simulink model "sps2se_pvinverter_avg"  (R2014a)
settings: Solver=ode15s  StartTime=0.0  StopTime=1  FixedStep=Ts  MaxStep=1e-3  RelTol=1e-4
PreLoadFcn:
  | PVArrayIsc = 5;
  | PVArrayVoc = 21.6;
  | PVArrayRs = 0.036;
  | Tcircuit = 27.15;
  | Toffset = -2;
  | TIPH1 = 0.001;
  | TXIS1 = 3;
  | TRS1 = 0;
  | Ts = 1e-4;
InitFcn:
  | Ts = 1e-4;
StartFcn:
  | tic;
StopFcn:
  | toc;
undefined symbols (not defined in the file or in its folder): sigbuilder_block
libraries: elec_lib x37, powerlib x9, nesl_utility x4, fl_lib x3, powerlib_meascontrol x1
settings Model: Creator=cosorio  LastModifiedBy=cosorio
settings DataIOCC: LimitDataPoints=off  SignalLoggingSaveFormat=ModelDataLogs  SaveOutput=off  SignalLogging=off  SaveTime=off
settings OptimizationCC: ExpressionDepthLimit=2147483647
settings DebuggingCC: UnderspecifiedInitializationDetection=Classic  SolverPrmCheckMsg=none  FcnCallInpInsideContextMsg=UseLocalSettings  StateNameClashWarn=warning
settings GRTTargetCC: CombineOutputUpdateFcns=off  GRTInterface=on

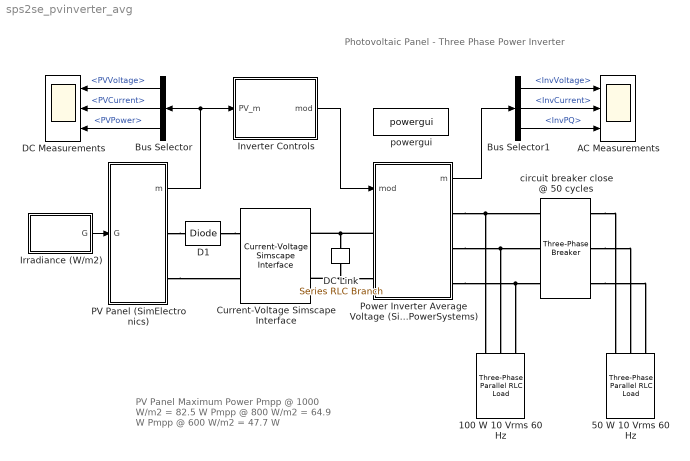
== system sps2se_pvinverter_avg ==
  note: Photovoltaic Panel - Three Phase Power Inverter
  note: PV Panel Maximum Power
      | Pmpp @ 1000 W/m2 = 82.5 W
      | Pmpp @ 800 W/m2 = 64.9 W
      | Pmpp @ 600 W/m2 = 47.7 W
  100 W 10 Vrms 60 Hz : powerlib/Elements/Three-Phase Parallel RLC Load  LConnTagsString=A|B|C  Configuration=Y (grounded)  NominalVoltage=10  NominalFrequency=60  ActivePower=100  InductivePower=0  CapacitivePower=0  Measurements=None  LoadType=constant Z
  50 W 10 Vrms 60 Hz : powerlib/Elements/Three-Phase Parallel RLC Load  LConnTagsString=A|B|C  Configuration=Y (grounded)  NominalVoltage=10  NominalFrequency=60  ActivePower=50  InductivePower=0  CapacitivePower=0  Measurements=None  LoadType=constant Z
  AC Measurements : Scope  NumInputPorts=3
      settings: YMin=-10~-10~0  YMax=10~10~100  SaveName=InverterData
  Bus Selector : BusSelector  OutputSignals=PVVoltage,PVCurrent,PVPower
  Bus Selector1 : BusSelector  OutputSignals=InvVoltage,InvCurrent,InvPQ
  Current-Voltage Simscape Interface : powerlib/Interface Elements/Current-Voltage Simscape Interface  DFT=off  FMode=Unit delay (discrete)  T=1e-4  Ts=1e-4  i0=0  v0=18  Sd=SimPowerSystems side  Measurements=off
  D1 : elec_lib/Semiconductor Devices/Diode  ModelType=3  Vf=0.6 V  Ron=0.3 Ohm  Goff=1e-8 S  Rz=0.3 Ohm  Vz=50 V  C_PWL=5 pF  prmExp=1  I12=[ 0.0137 0.545 ] A  V12=[ 0.6 0.7 ] V  I1=0.0137 A  V1=0.6 V  RS=0.01 Ohm  IS=1e-12 A  Tmeas=25 C  ec=1  BV=Inf V  C_param=1  CJ0=5 pF  VJ=1 V  Mgrad=0.5  Vvec=[ 0.1 10 100 ] V  Cvec=[ 3.5 1 0.4 ] pF  FC=0.5  Q_param=1  Irrm=-7.15 A  iF=4 A  didt=-750 A/us  trr=115 ns  TT=50 ns  tau=100 ns  T_param=1  IS_T2=1.25e-7 A  I1_T2=0.245 A  V1_T2=0.5 V  Tmeas2=125 C  EG_param=1  EG=1.11 eV  XTI_param=1  XTI=3  dBVdT=0 V/K  Tdevice=25 C  Rth=[ 0 10 ] K/W  thermal_mass_parameterization=1  thermal_mass=[ 0 1 ] J/K  thermal_time_constant=[ 0 10 ] s  thermal_mass_initial_temperatures=[ 25 25 ] C
  DC Link : powerlib/Elements/Series RLC Branch  LConnTagsString=__new0  RConnTagsString=__new0  BranchType=C  Resistance=1  Inductance=1e-3  SetiL0=off  InitialCurrent=0  Capacitance=480e-6  Setx0=on  InitialVoltage=18  Measurements=None
  DC Measurements : Scope  NumInputPorts=3
      settings: YMin=0~0~0  YMax=25~6~100
  Inverter Controls : Subsystem  TreatAsAtomicUnit=on  SystemSampleTime=1e-4
  Irradiance (W/m2) : Subsystem  Tag=STV Subsys  LoadFcn=sigbuilder_block('load');  StartFcn=sigbuilder_block('start');  StopFcn=sigbuilder_block('stop');  ClipboardFcn=sigbuilder_block('clipboard');  mask(Sigbuilder block){}
      mask help: Sigbuilder GUI
      mask init:
      | if ~strcmp(get_param(bdroot(gcbh),'SimulationStatus'),'stopped') tuvar = sigbuilder_block('maskInit'); end
      settings: CopyFcn=sigbuilder_block('copy');  DeleteFcn=sigbuilder_block('delete');  ModelCloseFcn=sigbuilder_block('modelClose');  PreSaveFcn=sigbuilder_block('preSave');  PauseFcn=sigbuilder_block('pause')  ContinueFcn=sigbuilder_block('continue')  NameChangeFcn=sigbuilder_block('namechange');  OpenFcn=sigbuilder_block('open',[124.138 46.5517 550.552 391.034 ]);  CloseFcn=sigbuilder_block('close');
      mask Display: plot(0,0,100,100,[10,10,40,40,10],[80,20,20,80,80],[40,10],[50,50], [40,27,10],[65,72,56],[40,25,25,10],[28,28,43,43]);
  PV Panel (SimElectronics) : Subsystem
  Power Inverter Average Voltage (SimPowerSystems) : Subsystem
  circuit breaker close @ 50 cycles : powerlib/Elements/Three-Phase Breaker  InitialState=open  SwitchA=on  SwitchB=on  SwitchC=on  SwitchTimes=[50/60]  External=off  BreakerResistance=0.001  SnubberResistance=1e6  SnubberCapacitance=inf  Measurements=None
  powergui : powerlib/powergui  Priority=1  SimulationMode=Discrete  SolverType=Tustin  SampleTime=Ts  frequency=60  SPID=off  DisableSnubberDevices=off  DisableRonSwitches=off  DisableVfSwitches=off  SwTol=0  Interpol=off  DisplayEquations=off  Ts=0  methode=off  frequencyindice=0  Pbase=100e6  ErrMax=1e-4  Iterations=50  UnitsV=kV  UnitsW=MW  FunctionMessages=off  echomessages=off  HookPort=off  EnableUseOfTLC=off  x0status=blocks  RestoreLinks=warning  ResistiveCurrentMeasurement=off  Frange=[0:2:500]  Ylog=off  Xlog=on  ShowGrid=off  save=off  variable=ZData  structure=0  ZoomFFT=on  StartTime=0.0  cycles=1  DisplayStyle=1  fundamental=60  FreqAxis=off  MaxFrequency=1000  frequencyindicesteady=1  RmsSteady=1  display=off
  wires:
  Irradiance (W/m2)/1(G) -> PV Panel (SimElectronics)/1(G)
  PV Panel (SimElectronics)/1(m) -> Bus Selector/1, Inverter Controls/1(PV_m)
  Bus Selector/3 -> DC Measurements/3  "<PVPower>"
  Bus Selector/1 -> DC Measurements/1  "<PVVoltage>"
  Bus Selector/2 -> DC Measurements/2  "<PVCurrent>"
  Power Inverter Average Voltage (SimPowerSystems)/1(m) -> Bus Selector1/1
  Bus Selector1/1 -> AC Measurements/1  "<InvVoltage>"
  Bus Selector1/2 -> AC Measurements/2  "<InvCurrent>"
  Bus Selector1/3 -> AC Measurements/3  "<InvPQ>"
  Inverter Controls/1(mod) -> Power Inverter Average Voltage (SimPowerSystems)/1(mod)
  connections:
  PV Panel (SimElectronics)/RConn2 -- Current-Voltage Simscape Interface/RConn2
  DC Link/RConn1 -- Current-Voltage Simscape Interface/LConn2 -- Power Inverter Average Voltage (SimPowerSystems)/LConn2
  Power Inverter Average Voltage (SimPowerSystems)/LConn1 -- Current-Voltage Simscape Interface/LConn1 -- DC Link/LConn1
  PV Panel (SimElectronics)/RConn1 -- D1/LConn1
  D1/RConn1 -- Current-Voltage Simscape Interface/RConn1
  Power Inverter Average Voltage (SimPowerSystems)/RConn1 -- 100 W 10 Vrms 60 Hz/LConn1 -- circuit breaker close @ 50 cycles/LConn1
  Power Inverter Average Voltage (SimPowerSystems)/RConn3 -- 100 W 10 Vrms 60 Hz/LConn3 -- circuit breaker close @ 50 cycles/LConn3
  Power Inverter Average Voltage (SimPowerSystems)/RConn2 -- 100 W 10 Vrms 60 Hz/LConn2 -- circuit breaker close @ 50 cycles/LConn2
  circuit breaker close @ 50 cycles/RConn1 -- 50 W 10 Vrms 60 Hz/LConn1
  circuit breaker close @ 50 cycles/RConn2 -- 50 W 10 Vrms 60 Hz/LConn2
  circuit breaker close @ 50 cycles/RConn3 -- 50 W 10 Vrms 60 Hz/LConn3

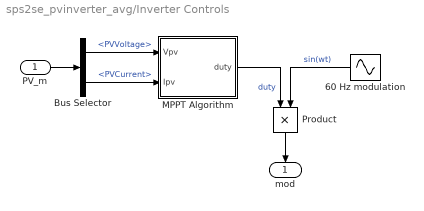
== system sps2se_pvinverter_avg/Inverter Controls ==
  PV_m : Inport
  60 Hz modulation : Sin  Frequency=2*pi*60  Phase=[0, 120*pi/180, -120*pi/180]  SampleTime=1e-4
  Bus Selector : BusSelector  OutputSignals=PVVoltage,PVCurrent
  MPPT Algorithm : Subsystem
  Product : Product  RndMeth=Zero
  mod : Outport
  wires:
  60 Hz modulation/1 -> Product/2  "sin(wt)"
  PV_m/1 -> Bus Selector/1
  Product/1 -> mod/1
  Bus Selector/1 -> MPPT Algorithm/1(Vpv)  "<PVVoltage>"
  Bus Selector/2 -> MPPT Algorithm/2(Ipv)  "<PVCurrent>"
  MPPT Algorithm/1(duty) -> Product/1  "duty"

== system sps2se_pvinverter_avg/Irradiance (W//m2) ==
  Demux : Demux  Tag=STV Demux  Outputs=1
  FromWs : FromWorkspace  Tag=STV FromWs  VariableName=tuvar  SampleTime=0
      SigBuilderData=|
      | common.afterFinalStr = 'Extrapolate'
      | common.sampleTime = '0'
      | dataSet(1).timeRange = [0 1]
      | dataSet(1).name = 'Constant Irradiance'
      | dataSet(2).timeRange = [0 1]
      | dataSet(2).name = 'Step Irradiance'
      | dataSet(3).timeRange = [0 1]
      | dataSet(3).name = 'Trapezoidal Irradiance'
      | sbobj.Groups(1).Name = 'Constant Irradiance'
      | sbobj.Groups(1).Signals.Name = 'G'
      | sbobj.Groups(1).Signals.XData = [0 1]
      | sbobj.Groups(1).Signals.YData = [800 800]
      | sbobj.Groups(1).TimeRange = [0 1]
      | sbobj.Groups(2).Name = 'Step Irradiance'
      | sbobj.Groups(2).Signals.Name = 'G'
      | sbobj.Groups(2).Signals.XData = [0 0.5 0.5 1]
      | sbobj.Groups(2).Signals.YData = [600 600 1000 1000]
      | sbobj.Groups(2).TimeRange = [0 1]
      | sbobj.Groups(3).Name = 'Trapezoidal Irradiance'
      | sbobj.Groups(3).Signals.Name = 'G'
      | sbobj.Groups(3).Signals.XData = [0 0.2 0.3 0.5 0.7 0.9 1]
      | sbobj.Groups(3).Signals.YData = [800 800 600 600 1000 1000 800]
      | sbobj.Groups(3).TimeRange = [0 1]
  G : Outport  Tag=STV Outport
  wires:
  Demux/1 -> G/1
  FromWs/1 -> Demux/1

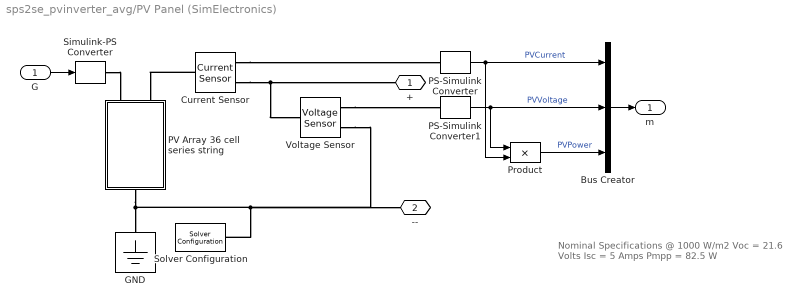
== system sps2se_pvinverter_avg/PV Panel (SimElectronics) ==
  note: Nominal Specifications @ 1000 W/m2
      | Voc = 21.6 Volts
      | Isc = 5 Amps
      | Pmpp = 82.5 W
  G : Inport
  Bus Creator : BusCreator  Inputs=3
  Current Sensor : fl_lib/Electrical/Electrical Sensors/Current Sensor
  GND : fl_lib/Electrical/Electrical Elements/Electrical Reference
  PS-Simulink Converter : nesl_utility/PS-Simulink Converter  PhysicalDomain=network_engine_domain  SubClassName=ps_output  LeftPortType=input  RightPortType=output  PseudoPeriodic=off  Frequencies=[]  Unit=A  AffineConversion=off
  PS-Simulink Converter1 : nesl_utility/PS-Simulink Converter  PhysicalDomain=network_engine_domain  SubClassName=ps_output  LeftPortType=input  RightPortType=output  PseudoPeriodic=off  Frequencies=[]  Unit=V  AffineConversion=off
  PV Array 36 cell series string : Subsystem
  Product : Product  RndMeth=Zero
  Simulink-PS Converter : nesl_utility/Simulink-PS Converter  PhysicalDomain=network_engine_domain  SubClassName=ps_input  LeftPortType=input  RightPortType=output  PseudoPeriodic=off  Frequencies=[]  NoiseDistribution=none  NoiseParameters=[]  Unit=W/m^2  AffineConversion=off  InputFiltering=off  SimscapeFilterOrder=1  InputFilterTimeConstant=1e-4  UdotUserProvided=0
  Solver Configuration : nesl_utility/Solver Configuration  PhysicalDomain=network_engine_domain  SubClassName=solver  LeftPortType=input  RightPortType=generic  Accelerate=off  Tones=[]  Harmonics=[]  SimulateNoise=off  Profile=off  UseLocalSampling=off  EnableSwitchedLinearOptims=on  FrequencyDomain=off  UseCCode=off  RelTol=0.001  AbsTol=1e-06  MinStep=1e-09  ToWorkspace=off  DoDC=on  ResidualTolerance=1e-9  UseLocalSolver=on  LocalSolverChoice=NE_BACKWARD_EULER_ADVANCER  LocalSolverSampleTime=1e-4  DoFixedCost=on  MaxNonlinIter=4  MaxModeIter=2  LinearAlgebra=Sparse  DelaysMemoryBudget=1024  AutomaticFiltering=on  FilteringTimeConstant=0.001
  Voltage Sensor : fl_lib/Electrical/Electrical Sensors/Voltage Sensor
  + : PMIOPort  Port=1  Side=Right
  -- : PMIOPort  Port=2  Side=Right
  m : Outport
  wires:
  G/1 -> Simulink-PS Converter/1
  PS-Simulink Converter/1 -> Bus Creator/1, Product/2  "PVCurrent"
  PS-Simulink Converter1/1 -> Bus Creator/2, Product/1  "PVVoltage"
  Bus Creator/1 -> m/1
  Product/1 -> Bus Creator/3  "PVPower"
  connections:
  --/RConn1 -- Voltage Sensor/RConn2 -- Solver Configuration/RConn1 -- PV Array 36 cell series string/RConn1 -- GND/LConn1
  Simulink-PS Converter/RConn1 -- PV Array 36 cell series string/LConn1
  Current Sensor/LConn1 -- PV Array 36 cell series string/LConn2
  Current Sensor/RConn2 -- +/RConn1 -- Voltage Sensor/LConn1
  Current Sensor/RConn1 -- PS-Simulink Converter/LConn1
  Voltage Sensor/RConn1 -- PS-Simulink Converter1/LConn1

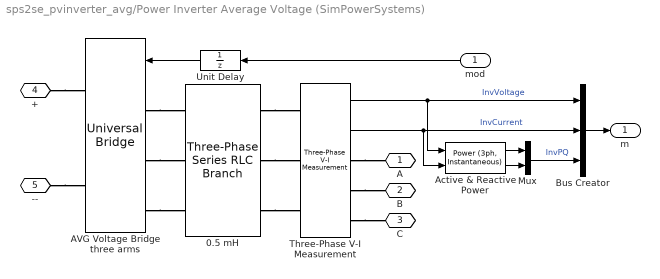
== system sps2se_pvinverter_avg/Power Inverter Average Voltage (SimPowerSystems) ==
  mod : Inport
  0.5 mH : powerlib/Elements/Three-Phase Series RLC Branch  LConnTagsString=A|B|C  RConnTagsString=A|B|C  BranchType=L  Resistance=1.0  Inductance=500e-6  Capacitance=1.0  Measurements=None
  AVG Voltage Bridge three arms : powerlib/Power Electronics/Universal Bridge  Arms=3  SnubberResistance=1e5  SnubberCapacitance=inf  Device=Average-model based VSC  Ron=1e-3  Lon=0  ForwardVoltages="[  0  0  ]"  ForwardVoltage=0  GTOparameters=[ 10e-6 , 20e-6 ]  IGBTparameters=[ 1e-6 , 2e-6 ]  Measurements=None  Measurements_2=None  converterType=Rectifier
  Active & Reactive Power : powerlib_meascontrol/Measurements/Power (3ph, Instantaneous)
  Bus Creator : BusCreator  Inputs=3
  Mux : Mux  Inputs=2
  Three-Phase V-I Measurement : powerlib/Measurements/Three-Phase V-I Measurement  VoltageMeasurement=phase-to-ground  SetLabelV=off  LabelV=Vabc  Vpu=off  VpuLL=off  CurrentMeasurement=yes  SetLabelI=off  LabelI=Iabc  Ipu=off  Pbase=100e6  Vbase=500e3  OutputType=Complex  PhasorSimulation=off  PSBequivalent=0
  Unit Delay : UnitDelay  SampleTime=Ts
  A : PMIOPort  Port=1  Side=Right
  B : PMIOPort  Port=2  Side=Right
  C : PMIOPort  Port=3  Side=Right
  + : PMIOPort  Port=4  Side=Left
  -- : PMIOPort  Port=5  Side=Left
  m : Outport
  wires:
  Three-Phase V-I Measurement/1 -> Bus Creator/1, Active & Reactive Power/1  "InvVoltage"
  Mux/1 -> Bus Creator/3  "InvPQ"
  Three-Phase V-I Measurement/2 -> Bus Creator/2, Active & Reactive Power/2  "InvCurrent"
  Bus Creator/1 -> m/1
  mod/1 -> Unit Delay/1
  Unit Delay/1 -> AVG Voltage Bridge three arms/1
  Active & Reactive Power/2 -> Mux/2
  Active & Reactive Power/1 -> Mux/1
  connections:
  AVG Voltage Bridge three arms/LConn1 -- 0.5 mH/LConn1
  AVG Voltage Bridge three arms/LConn2 -- 0.5 mH/LConn2
  AVG Voltage Bridge three arms/LConn3 -- 0.5 mH/LConn3
  0.5 mH/RConn1 -- Three-Phase V-I Measurement/LConn1
  0.5 mH/RConn2 -- Three-Phase V-I Measurement/LConn2
  0.5 mH/RConn3 -- Three-Phase V-I Measurement/LConn3
  Three-Phase V-I Measurement/RConn1 -- A/RConn1
  Three-Phase V-I Measurement/RConn2 -- B/RConn1
  Three-Phase V-I Measurement/RConn3 -- C/RConn1
  +/RConn1 -- AVG Voltage Bridge three arms/RConn1
  --/RConn1 -- AVG Voltage Bridge three arms/RConn2

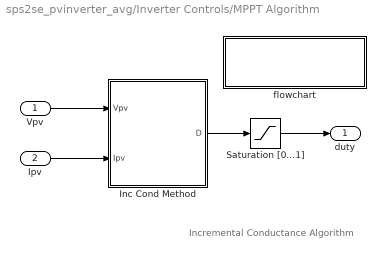
== system sps2se_pvinverter_avg/Inverter Controls/MPPT Algorithm ==
  note: Incremental Conductance Algorithm
  Vpv : Inport  OutDataTypeStr=double  PortDimensions=1  SampleTime=[0.0001,0]
  Ipv : Inport  Port=2  OutDataTypeStr=double  PortDimensions=1  SampleTime=[0.0001,0]
  Inc Cond Method : Stateflow chart  TreatAsAtomicUnit=on
  Saturation [0...1] : Saturate  UpperLimit=1  LowerLimit=0
  flowchart : Subsystem
      settings: OpenFcn=winopen('INC.jpg');
      mask Display: disp('Algorithm\nFlowchart')
  duty : Outport  OutDataTypeStr=double  PortDimensions=1  SampleTime=[0.0001,0]
  wires:
  Inc Cond Method/1(D) -> Saturation [0...1]/1
  Vpv/1 -> Inc Cond Method/1(Vpv)
  Ipv/1 -> Inc Cond Method/2(Ipv)
  Saturation [0...1]/1 -> duty/1

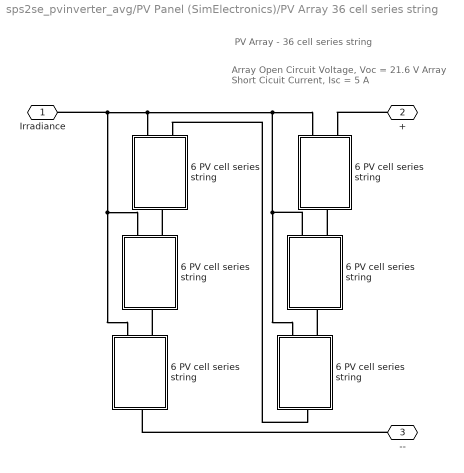
== system sps2se_pvinverter_avg/PV Panel (SimElectronics)/PV Array 36 cell series string ==
  note: Array Open Circuit Voltage, Voc = 21.6 V
      | Array Short Cicuit Current, Isc = 5 A
  note: PV Array - 36 cell series string
  6 PV cell series string : Subsystem  mask(PV String){Isc=PVArrayIsc, Voc=PVArrayVoc/6, N=1.5, Rs=PVArrayRs/6, TIPH1=TIPH1, TXIS1=TXIS1, TRS1=TRS1, TOFFSET=Toffset}
      mask prompts: Isc "Short-circuit current (A) :"; Voc "Open-circuit voltage (V) :"; N "Quality factor :"; Rs "Series resistance (ohms) :"; TIPH1 "1st order temperature coefficient for solar generated current (1/oC) :"; TXIS1 "Temperature exponent for diode saturation current :"; TRS1 "Temperature exponent for series resistance :"; TOFFSET "Offset local circuit temperature (oC) :"
      mask help:
      | PV series string.
      | This block models six (6) photo-voltaic cells connected in series.
      | The base parameters are measured at an irradiance of 1000 W/m2 and a device
      | temperature of 25oC.
      | The string short-circuit current is equal to the short-circuit current of each
      | individual cell.
      | The string open-circuit voltage is equal to six times the open-circuit voltage
      | of each individual cell.
      | The string series resistance is equal to six times the series resistance of
      | each individual cell.
      | The offset local circuit temperature is the difference between the string
      | temperature and the specified circuit temperature.
  "6 PV cell series string " : Subsystem  mask(PV String){Isc=PVArrayIsc, Voc=PVArrayVoc/6, N=1.5, Rs=PVArrayRs/6, TIPH1=TIPH1, TXIS1=TXIS1, TRS1=TRS1, TOFFSET=Toffset}
      mask prompts: Isc "Short-circuit current (A) :"; Voc "Open-circuit voltage (V) :"; N "Quality factor :"; Rs "Series resistance (ohms) :"; TIPH1 "1st order temperature coefficient for solar generated current (1/oC) :"; TXIS1 "Temperature exponent for diode saturation current :"; TRS1 "Temperature exponent for series resistance :"; TOFFSET "Offset local circuit temperature (oC) :"
      mask help:
      | PV series string.
      | This block models six (6) photo-voltaic cells connected in series.
      | The base parameters are measured at an irradiance of 1000 W/m2 and a device
      | temperature of 25oC.
      | The string short-circuit current is equal to the short-circuit current of each
      | individual cell.
      | The string open-circuit voltage is equal to six times the open-circuit voltage
      | of each individual cell.
      | The string series resistance is equal to six times the series resistance of
      | each individual cell.
      | The offset local circuit temperature is the difference between the string
      | temperature and the specified circuit temperature.
  "6 PV cell series string  " : Subsystem  mask(PV String){Isc=PVArrayIsc, Voc=PVArrayVoc/6, N=1.5, Rs=PVArrayRs/6, TIPH1=TIPH1, TXIS1=TXIS1, TRS1=TRS1, TOFFSET=Toffset}
      mask prompts: Isc "Short-circuit current (A) :"; Voc "Open-circuit voltage (V) :"; N "Quality factor :"; Rs "Series resistance (ohms) :"; TIPH1 "1st order temperature coefficient for solar generated current (1/oC) :"; TXIS1 "Temperature exponent for diode saturation current :"; TRS1 "Temperature exponent for series resistance :"; TOFFSET "Offset local circuit temperature (oC) :"
      mask help:
      | PV series string.
      | This block models six (6) photo-voltaic cells connected in series.
      | The base parameters are measured at an irradiance of 1000 W/m2 and a device
      | temperature of 25oC.
      | The string short-circuit current is equal to the short-circuit current of each
      | individual cell.
      | The string open-circuit voltage is equal to six times the open-circuit voltage
      | of each individual cell.
      | The string series resistance is equal to six times the series resistance of
      | each individual cell.
      | The offset local circuit temperature is the difference between the string
      | temperature and the specified circuit temperature.
  "6 PV cell series string   " : Subsystem  mask(PV String){Isc=PVArrayIsc, Voc=PVArrayVoc/6, N=1.5, Rs=PVArrayRs/6, TIPH1=TIPH1, TXIS1=TXIS1, TRS1=TRS1, TOFFSET=Toffset}
      mask prompts: Isc "Short-circuit current (A) :"; Voc "Open-circuit voltage (V) :"; N "Quality factor :"; Rs "Series resistance (ohms) :"; TIPH1 "1st order temperature coefficient for solar generated current (1/oC) :"; TXIS1 "Temperature exponent for diode saturation current :"; TRS1 "Temperature exponent for series resistance :"; TOFFSET "Offset local circuit temperature (oC) :"
      mask help:
      | PV series string.
      | This block models six (6) photo-voltaic cells connected in series.
      | The base parameters are measured at an irradiance of 1000 W/m2 and a device
      | temperature of 25oC.
      | The string short-circuit current is equal to the short-circuit current of each
      | individual cell.
      | The string open-circuit voltage is equal to six times the open-circuit voltage
      | of each individual cell.
      | The string series resistance is equal to six times the series resistance of
      | each individual cell.
      | The offset local circuit temperature is the difference between the string
      | temperature and the specified circuit temperature.
  "6 PV cell series string    " : Subsystem  mask(PV String){Isc=PVArrayIsc, Voc=PVArrayVoc/6, N=1.5, Rs=PVArrayRs/6, TIPH1=TIPH1, TXIS1=TXIS1, TRS1=TRS1, TOFFSET=Toffset}
      mask prompts: Isc "Short-circuit current (A) :"; Voc "Open-circuit voltage (V) :"; N "Quality factor :"; Rs "Series resistance (ohms) :"; TIPH1 "1st order temperature coefficient for solar generated current (1/oC) :"; TXIS1 "Temperature exponent for diode saturation current :"; TRS1 "Temperature exponent for series resistance :"; TOFFSET "Offset local circuit temperature (oC) :"
      mask help:
      | PV series string.
      | This block models six (6) photo-voltaic cells connected in series.
      | The base parameters are measured at an irradiance of 1000 W/m2 and a device
      | temperature of 25oC.
      | The string short-circuit current is equal to the short-circuit current of each
      | individual cell.
      | The string open-circuit voltage is equal to six times the open-circuit voltage
      | of each individual cell.
      | The string series resistance is equal to six times the series resistance of
      | each individual cell.
      | The offset local circuit temperature is the difference between the string
      | temperature and the specified circuit temperature.
  "6 PV cell series string     " : Subsystem  mask(PV String){Isc=PVArrayIsc, Voc=PVArrayVoc/6, N=1.5, Rs=PVArrayRs/6, TIPH1=TIPH1, TXIS1=TXIS1, TRS1=TRS1, TOFFSET=Toffset}
      mask prompts: Isc "Short-circuit current (A) :"; Voc "Open-circuit voltage (V) :"; N "Quality factor :"; Rs "Series resistance (ohms) :"; TIPH1 "1st order temperature coefficient for solar generated current (1/oC) :"; TXIS1 "Temperature exponent for diode saturation current :"; TRS1 "Temperature exponent for series resistance :"; TOFFSET "Offset local circuit temperature (oC) :"
      mask help:
      | PV series string.
      | This block models six (6) photo-voltaic cells connected in series.
      | The base parameters are measured at an irradiance of 1000 W/m2 and a device
      | temperature of 25oC.
      | The string short-circuit current is equal to the short-circuit current of each
      | individual cell.
      | The string open-circuit voltage is equal to six times the open-circuit voltage
      | of each individual cell.
      | The string series resistance is equal to six times the series resistance of
      | each individual cell.
      | The offset local circuit temperature is the difference between the string
      | temperature and the specified circuit temperature.
  Irradiance : PMIOPort  Port=1  Side=Left
  + : PMIOPort  Port=2  Side=Left
  -- : PMIOPort  Port=3  Side=Right
  connections:
  "6 PV cell series string    "/LConn1 -- "6 PV cell series string     "/LConn1 -- Irradiance/RConn1 -- "6 PV cell series string  "/LConn1 -- "6 PV cell series string "/LConn1 -- 6 PV cell series string/LConn1 -- "6 PV cell series string   "/LConn1
  --/RConn1 -- "6 PV cell series string     "/RConn1
  +/RConn1 -- 6 PV cell series string/LConn2
  "6 PV cell series string     "/LConn2 -- "6 PV cell series string    "/RConn1
  "6 PV cell series string    "/LConn2 -- "6 PV cell series string   "/RConn1
  "6 PV cell series string  "/RConn1 -- "6 PV cell series string   "/LConn2
  "6 PV cell series string  "/LConn2 -- "6 PV cell series string "/RConn1
  "6 PV cell series string "/LConn2 -- 6 PV cell series string/RConn1

== system sps2se_pvinverter_avg/Inverter Controls/MPPT Algorithm/flowchart ==

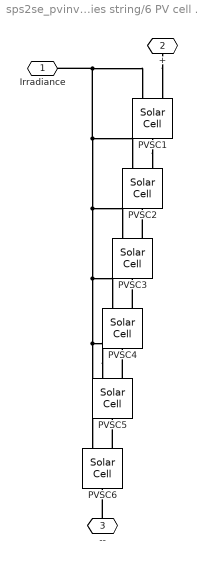
== system sps2se_pvinverter_avg/PV Panel (SimElectronics)/PV Array 36 cell series string/6 PV cell series string ==
  PVSC{1..6} (6 alike) : elec_lib/Sources/Solar Cell  prm=1  Isc=Isc A  Voc=Voc/6 V  Is=1e-06 A  Is2=0 A  Iph=7.34 A  Ir0=1000 W/m^2  ec=N  N2=2  Rs=Rs/6 Ohm  Rp=Inf Ohm  N_series=1  TIPH1=TIPH1 1/K  EG=1.11 eV  TXIS1=TXIS1  TXIS2=3  TRS1=TRS1  TRP1=0  Tmeas=25 C  TFIXED=25 C  thermal_mass=100 J/K  initial_temperature=25 C
  Irradiance : PMIOPort  Port=1  Side=Left
  + : PMIOPort  Port=2  Side=Left
  -- : PMIOPort  Port=3  Side=Right
  connections:
  --/RConn1 -- PVSC6/RConn1
  +/RConn1 -- PVSC1/LConn2
  PVSC6/LConn2 -- PVSC5/RConn1
  PVSC5/LConn2 -- PVSC4/RConn1
  PVSC4/LConn2 -- PVSC3/RConn1
  PVSC3/LConn2 -- PVSC2/RConn1
  PVSC1/RConn1 -- PVSC2/LConn2
  PVSC5/LConn1 -- PVSC4/LConn1 -- PVSC3/LConn1 -- PVSC2/LConn1 -- PVSC1/LConn1 -- Irradiance/RConn1 -- PVSC6/LConn1

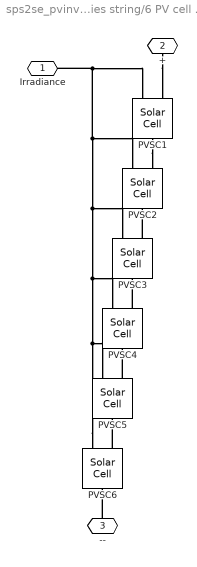
== system sps2se_pvinverter_avg/PV Panel (SimElectronics)/PV Array 36 cell series string/6 PV cell series string  ==
  PVSC{1..6} (6 alike) : elec_lib/Sources/Solar Cell  prm=1  Isc=Isc A  Voc=Voc/6 V  Is=1e-06 A  Is2=0 A  Iph=7.34 A  Ir0=1000 W/m^2  ec=N  N2=2  Rs=Rs/6 Ohm  Rp=Inf Ohm  N_series=1  TIPH1=TIPH1 1/K  EG=1.11 eV  TXIS1=TXIS1  TXIS2=3  TRS1=TRS1  TRP1=0  Tmeas=25 C  TFIXED=25 C  thermal_mass=100 J/K  initial_temperature=25 C
  Irradiance : PMIOPort  Port=1  Side=Left
  + : PMIOPort  Port=2  Side=Left
  -- : PMIOPort  Port=3  Side=Right
  connections:
  PVSC6/LConn1 -- Irradiance/RConn1 -- PVSC1/LConn1 -- PVSC2/LConn1 -- PVSC3/LConn1 -- PVSC4/LConn1 -- PVSC5/LConn1
  PVSC1/RConn1 -- PVSC2/LConn2
  PVSC3/LConn2 -- PVSC2/RConn1
  PVSC4/LConn2 -- PVSC3/RConn1
  PVSC5/LConn2 -- PVSC4/RConn1
  PVSC6/LConn2 -- PVSC5/RConn1
  +/RConn1 -- PVSC1/LConn2
  --/RConn1 -- PVSC6/RConn1

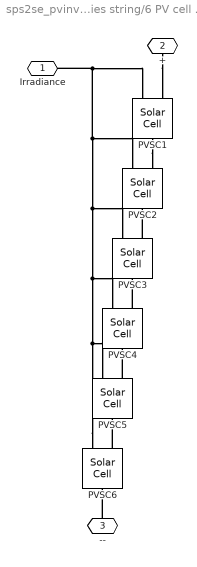
== system sps2se_pvinverter_avg/PV Panel (SimElectronics)/PV Array 36 cell series string/6 PV cell series string   ==
  PVSC{1..6} (6 alike) : elec_lib/Sources/Solar Cell  prm=1  Isc=Isc A  Voc=Voc/6 V  Is=1e-06 A  Is2=0 A  Iph=7.34 A  Ir0=1000 W/m^2  ec=N  N2=2  Rs=Rs/6 Ohm  Rp=Inf Ohm  N_series=1  TIPH1=TIPH1 1/K  EG=1.11 eV  TXIS1=TXIS1  TXIS2=3  TRS1=TRS1  TRP1=0  Tmeas=25 C  TFIXED=25 C  thermal_mass=100 J/K  initial_temperature=25 C
  Irradiance : PMIOPort  Port=1  Side=Left
  + : PMIOPort  Port=2  Side=Left
  -- : PMIOPort  Port=3  Side=Right
  connections:
  PVSC6/LConn1 -- Irradiance/RConn1 -- PVSC1/LConn1 -- PVSC2/LConn1 -- PVSC3/LConn1 -- PVSC4/LConn1 -- PVSC5/LConn1
  PVSC1/RConn1 -- PVSC2/LConn2
  PVSC3/LConn2 -- PVSC2/RConn1
  PVSC4/LConn2 -- PVSC3/RConn1
  PVSC5/LConn2 -- PVSC4/RConn1
  PVSC6/LConn2 -- PVSC5/RConn1
  +/RConn1 -- PVSC1/LConn2
  --/RConn1 -- PVSC6/RConn1

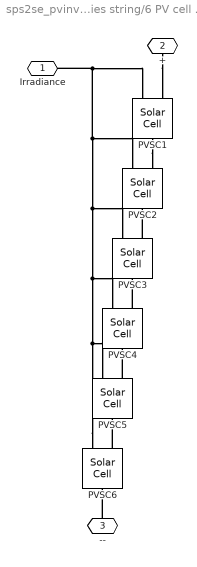
== system sps2se_pvinverter_avg/PV Panel (SimElectronics)/PV Array 36 cell series string/6 PV cell series string    ==
  PVSC{1..6} (6 alike) : elec_lib/Sources/Solar Cell  prm=1  Isc=Isc A  Voc=Voc/6 V  Is=1e-06 A  Is2=0 A  Iph=7.34 A  Ir0=1000 W/m^2  ec=N  N2=2  Rs=Rs/6 Ohm  Rp=Inf Ohm  N_series=1  TIPH1=TIPH1 1/K  EG=1.11 eV  TXIS1=TXIS1  TXIS2=3  TRS1=TRS1  TRP1=0  Tmeas=25 C  TFIXED=25 C  thermal_mass=100 J/K  initial_temperature=25 C
  Irradiance : PMIOPort  Port=1  Side=Left
  + : PMIOPort  Port=2  Side=Left
  -- : PMIOPort  Port=3  Side=Right
  connections:
  PVSC6/LConn1 -- Irradiance/RConn1 -- PVSC1/LConn1 -- PVSC2/LConn1 -- PVSC3/LConn1 -- PVSC4/LConn1 -- PVSC5/LConn1
  PVSC1/RConn1 -- PVSC2/LConn2
  PVSC3/LConn2 -- PVSC2/RConn1
  PVSC4/LConn2 -- PVSC3/RConn1
  PVSC5/LConn2 -- PVSC4/RConn1
  PVSC6/LConn2 -- PVSC5/RConn1
  +/RConn1 -- PVSC1/LConn2
  --/RConn1 -- PVSC6/RConn1

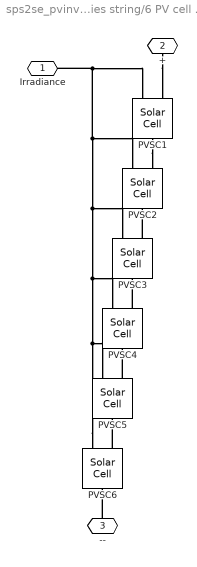
== system sps2se_pvinverter_avg/PV Panel (SimElectronics)/PV Array 36 cell series string/6 PV cell series string     ==
  PVSC{1..6} (6 alike) : elec_lib/Sources/Solar Cell  prm=1  Isc=Isc A  Voc=Voc/6 V  Is=1e-06 A  Is2=0 A  Iph=7.34 A  Ir0=1000 W/m^2  ec=N  N2=2  Rs=Rs/6 Ohm  Rp=Inf Ohm  N_series=1  TIPH1=TIPH1 1/K  EG=1.11 eV  TXIS1=TXIS1  TXIS2=3  TRS1=TRS1  TRP1=0  Tmeas=25 C  TFIXED=25 C  thermal_mass=100 J/K  initial_temperature=25 C
  Irradiance : PMIOPort  Port=1  Side=Left
  + : PMIOPort  Port=2  Side=Left
  -- : PMIOPort  Port=3  Side=Right
  connections:
  PVSC6/LConn1 -- Irradiance/RConn1 -- PVSC1/LConn1 -- PVSC2/LConn1 -- PVSC3/LConn1 -- PVSC4/LConn1 -- PVSC5/LConn1
  PVSC1/RConn1 -- PVSC2/LConn2
  PVSC3/LConn2 -- PVSC2/RConn1
  PVSC4/LConn2 -- PVSC3/RConn1
  PVSC5/LConn2 -- PVSC4/RConn1
  PVSC6/LConn2 -- PVSC5/RConn1
  +/RConn1 -- PVSC1/LConn2
  --/RConn1 -- PVSC6/RConn1

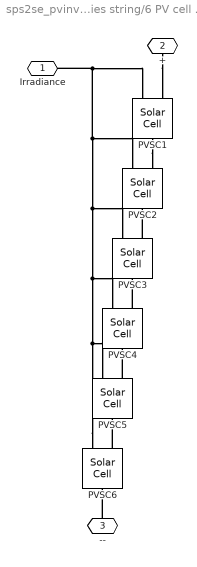
== system sps2se_pvinverter_avg/PV Panel (SimElectronics)/PV Array 36 cell series string/6 PV cell series string      ==
  PVSC{1..6} (6 alike) : elec_lib/Sources/Solar Cell  prm=1  Isc=Isc A  Voc=Voc/6 V  Is=1e-06 A  Is2=0 A  Iph=7.34 A  Ir0=1000 W/m^2  ec=N  N2=2  Rs=Rs/6 Ohm  Rp=Inf Ohm  N_series=1  TIPH1=TIPH1 1/K  EG=1.11 eV  TXIS1=TXIS1  TXIS2=3  TRS1=TRS1  TRP1=0  Tmeas=25 C  TFIXED=25 C  thermal_mass=100 J/K  initial_temperature=25 C
  Irradiance : PMIOPort  Port=1  Side=Left
  + : PMIOPort  Port=2  Side=Left
  -- : PMIOPort  Port=3  Side=Right
  connections:
  PVSC6/LConn1 -- Irradiance/RConn1 -- PVSC1/LConn1 -- PVSC2/LConn1 -- PVSC3/LConn1 -- PVSC4/LConn1 -- PVSC5/LConn1
  PVSC1/RConn1 -- PVSC2/LConn2
  PVSC3/LConn2 -- PVSC2/RConn1
  PVSC4/LConn2 -- PVSC3/RConn1
  PVSC5/LConn2 -- PVSC4/RConn1
  PVSC6/LConn2 -- PVSC5/RConn1
  +/RConn1 -- PVSC1/LConn2
  --/RConn1 -- PVSC6/RConn1

== stateflow chart sps2se_pvinverter_avg/Inverter Controls/MPPT Algorithm/Inc Cond Method ==
  settings: updateMethod=DISCRETE  sampleTime=1e-4
  state SAMPLEandCALCULATE
    entry:
    deltaV = Vpv - Vprev;
    deltaI = Ipv - Iprev;
    d = D;
  state INCREMENT_DUTY
    entry:
    d = d + deltad;
  state DECREMENT_DUTY
    entry:
    d = d - deltad;
  state RETURN
    entry:
    Vprev = Vpv; Iprev = Ipv;
    D = d;
  RETURN -> SAMPLEandCALCULATE
  (default) -> SAMPLEandCALCULATE
  SAMPLEandCALCULATE -> (junction 14) [order 1] : [deltaV > Vtol || deltaV < -Vtol]
  SAMPLEandCALCULATE -> (junction 15) [order 2]
  (junction 15) -> RETURN [order 3]
  (junction 15) -> INCREMENT_DUTY [order 1] : [deltaI < -Itol]
  (junction 14) -> RETURN [order 3]
  (junction 14) -> DECREMENT_DUTY [order 1] : [deltaI/deltaV > -Ipv/Vpv]
  (junction 14) -> INCREMENT_DUTY [order 2] : [deltaI/deltaV < -Ipv/Vpv]
  (junction 15) -> DECREMENT_DUTY [order 2] : [deltaI > Itol]
  INCREMENT_DUTY -> RETURN
  DECREMENT_DUTY -> RETURN
  data: Vpv input; Ipv input; D output double =0.8; Vprev local double =0; Iprev local double =0; Itol constant double =0.001; Vtol constant double =0.001; deltad constant double =0.0025; deltaV local double =0; deltaI local double =0; d local double =0
